simulink model "cps_stereo_analysis_v2"  (R2012b)
settings: Solver=FixedStepDiscrete  StartTime=0.0  StopTime=8.5  FixedStep=0.1  RelTol=1e-3  SampleTimeConstraint=STIndependent
libraries: visionutilities x3, visiongeotforms x3, visionstatistics x1, simulink x1
settings Model: RequirementInfo={} %GIDa_ba1ce617_85a9_495b_a3cb_2f0aceb7945f  MinMaxOverflowLogging=ForceOff  Creator=pmosterm  LastModifiedBy=pmosterm
settings SolverCC: EnableConcurrentExecution=on  ConcurrentTasks=on
settings DataIOCC: SignalLoggingSaveFormat=ModelDataLogs  SaveOutput=off  SaveTime=off
settings OptimizationCC: InlineParams=on
settings DebuggingCC: UnderspecifiedInitializationDetection=Simplified  FcnCallInpInsideContextMsg=EnableAllAsWarning  ModelReferenceExtraNoncontSigs=warning
settings ModelReferenceCC: ModelReferenceNumInstancesAllowed=Single
settings GRTTargetCC: CombineOutputUpdateFcns=off  GRTInterface=on
settings ConfigurationSet: Description=SimMechanics 2G

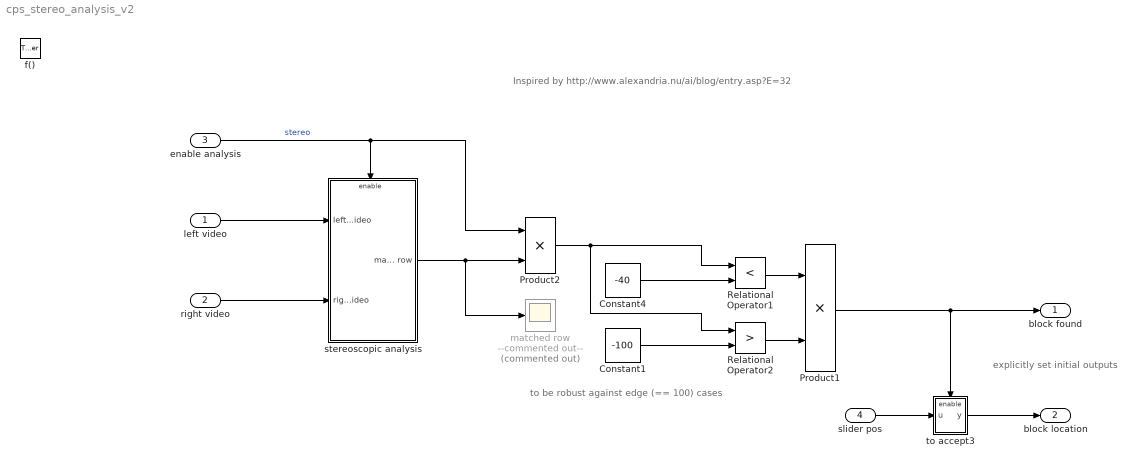
== system cps_stereo_analysis_v2 ==
  note: to be robust against
      | edge (== 100) cases
  note: Inspired by
      | http://www.alexandria.nu/ai/blog/entry.asp?E=32
  note: explicitly
      | set initial
      | outputs
  left video : Inport  OutDataTypeStr=uint8  PortDimensions=[400 240 3]
  right video : Inport  Port=2  OutDataTypeStr=uint8  PortDimensions=[400 240 3]
  enable analysis : Inport  Port=3  OutDataTypeStr=boolean  PortDimensions=1
  slider pos : Inport  Port=4  OutDataTypeStr=double  PortDimensions=1
  f() : TriggerPort  TriggerType=function-call  SampleTime=0.1  PortDimensions=1
  Constant1 : Constant  Value=-100  OutDataTypeStr=int16
  Constant4 : Constant  Value=-40  OutDataTypeStr=int16
  Product1 : Product  OutDataTypeStr=uint16  RndMeth=Zero
  Product2 : Product  RndMeth=Zero
  Relational Operator1 : RelationalOperator  Operator=<  OutDataTypeStr=fixdt(0,16)
  Relational Operator2 : RelationalOperator  Operator=>  OutDataTypeStr=fixdt(0,16)
  matched row --commented out-- : Scope  Commented=on
  stereoscopic analysis : Subsystem
  to accept3 : Subsystem  mask{yini=0}
      mask prompts: yini "Initial output"
      mask Display:
      | plot([1 2 3], [0 1 2]);
      | plot([1 2 3], [2 1 0]);
      | plot([5 6 7], [4 5 6]);
      | plot([5 6 7], [6 5 4]);
      | plot([9 10 11], [0 1 2]);
      | plot([9 10 11], [2 1 0]);
      | plot([0 6 6 12], [1 1 5 5]);
  block found : Outport  OutDataTypeStr=uint16  PortDimensions=1  InitialOutput=0
  block location : Outport  Port=2  OutDataTypeStr=double  PortDimensions=1  InitialOutput=0
  wires:
  left video/1 -> stereoscopic analysis/1(left video)
  enable analysis/1 -> Product2/1, stereoscopic analysis/Enable  "stereo"
  right video/1 -> stereoscopic analysis/2(right video)
  slider pos/1 -> to accept3/1(u)
  stereoscopic analysis/1(matched row) -> matched row --commented out--/1, Product2/2
  Constant4/1 -> Relational Operator1/2
  Product2/1 -> Relational Operator2/1, Relational Operator1/1
  to accept3/1(y) -> block location/1
  Constant1/1 -> Relational Operator2/2
  Relational Operator1/1 -> Product1/1
  Relational Operator2/1 -> Product1/2
  Product1/1 -> block found/1, to accept3/Enable

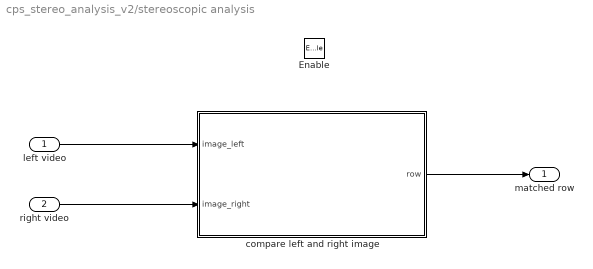
== system cps_stereo_analysis_v2/stereoscopic analysis ==
  left video : Inport
  right video : Inport  Port=2
  Enable : EnablePort
  compare left and right image : Subsystem  Variant=on  OverrideUsingVariant=textual
  matched row : Outport  InitialOutput=0
  wires:
  left video/1 -> compare left and right image/1(image_left)
  right video/1 -> compare left and right image/2(image_right)
  compare left and right image/1(row) -> matched row/1

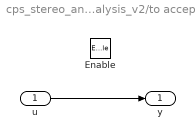
== system cps_stereo_analysis_v2/to accept3 ==
  u : Inport
  Enable : EnablePort
  y : Outport  InitialOutput=yini
  wires:
  u/1 -> y/1

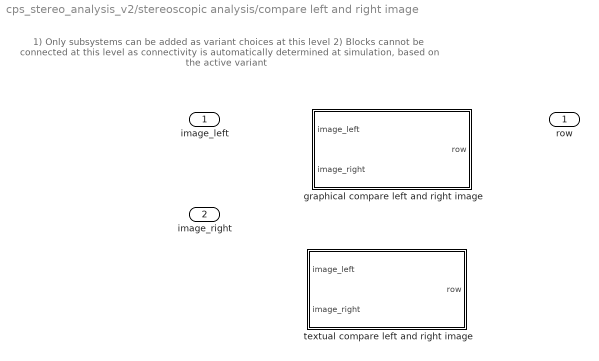
== system cps_stereo_analysis_v2/stereoscopic analysis/compare left and right image ==
  note: 1) Only subsystems can be added as variant choices at this level
      | 2) Blocks cannot be connected at this level as connectivity is
      | automatically determined at simulation, based on the active variant
  image_left : Inport
  image_right : Inport  Port=2
  graphical compare left and right image : Subsystem  VariantObject=graphical
  textual compare left and right image : MATLAB Function  TreatAsAtomicUnit=on  VariantObject=textual
  row : Outport

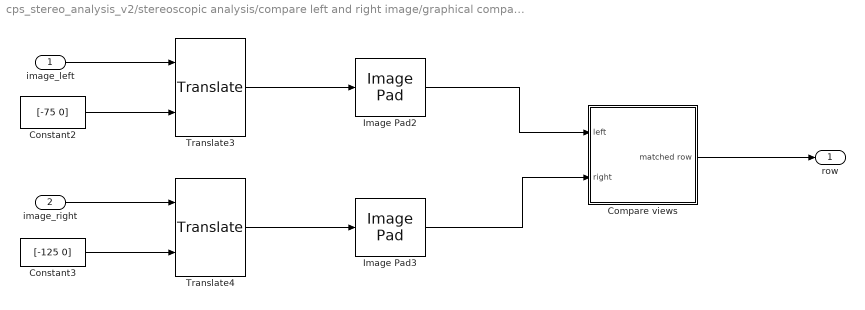
== system cps_stereo_analysis_v2/stereoscopic analysis/compare left and right image/graphical compare left and right image ==
  image_left : Inport
  image_right : Inport  Port=2
  Compare views : Subsystem  TreatAsAtomicUnit=on
  Constant2 : Constant  Value=[-75 0]  OutDataTypeStr=int16
  Constant3 : Constant  Value=[-125 0]  OutDataTypeStr=int16
  Image Pad2 : visionutilities/Image Pad  method=Constant  valSrc=Specify via dialog  value=0  spec=Output size  rowDirection=Right  outRowsMode=User-specified  rowSize=2  outColSize=120  colDirection=Bottom  outColsMode=User-specified  colSize=[60 80]  outRowSize=150  trunc_flag=None
  Image Pad3 : visionutilities/Image Pad  method=Constant  valSrc=Specify via dialog  value=0  spec=Output size  rowDirection=Right  outRowsMode=User-specified  rowSize=2  outColSize=120  colDirection=Bottom  outColsMode=User-specified  colSize=[60 80]  outRowSize=250  trunc_flag=None
  Translate3 : visiongeotforms/Translate  outSizeT=Same as input image  src_trans=Input port  translation="[1.5  2.3]"  maxOffset=[8 10]  fillVal=0  interpMethod=Bilinear  prodOutputMode=Binary point scaling  prodOutputWordLength=32  prodOutputFracLength=10  roundingMode=Nearest  overflowMode=on
  Translate4 : visiongeotforms/Translate  outSizeT=Same as input image  src_trans=Input port  translation="[1.5  2.3]"  maxOffset=[8 10]  fillVal=0  interpMethod=Bilinear  prodOutputMode=Binary point scaling  prodOutputWordLength=32  prodOutputFracLength=10  roundingMode=Nearest  overflowMode=on
  row : Outport
  wires:
  image_right/1 -> Translate4/1
  image_left/1 -> Translate3/1
  Constant2/1 -> Translate3/2
  Image Pad2/1 -> Compare views/1(left)
  Image Pad3/1 -> Compare views/2(right)
  Constant3/1 -> Translate4/2
  Translate3/1 -> Image Pad2/1
  Compare views/1(matched row) -> row/1
  Translate4/1 -> Image Pad3/1

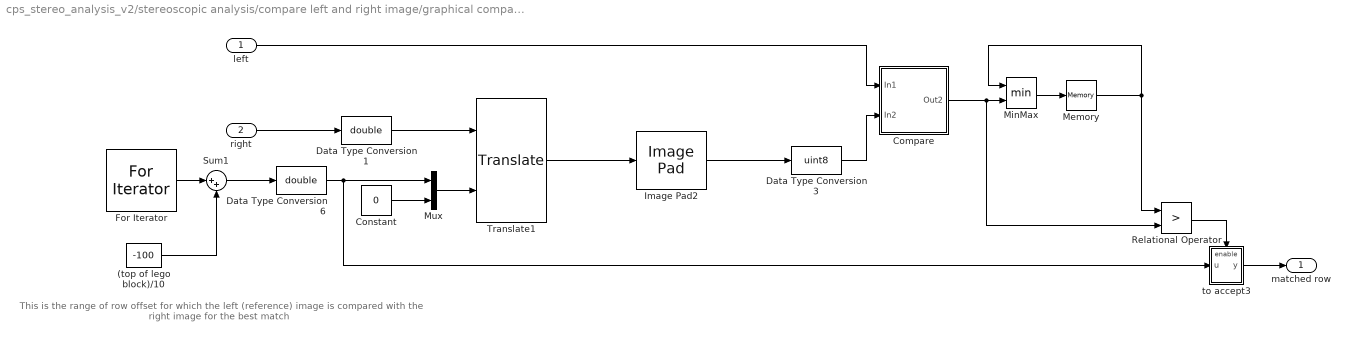
== system cps_stereo_analysis_v2/stereoscopic analysis/compare left and right image/graphical compare left and right image/Compare views ==
  note: This is the range of
      | row offset for which the
      | left (reference) image
      | is compared with the
      | right image for the
      | best match
  left : Inport
  right : Inport  Port=2
  (top of lego block)/10 : Constant  Value=-100
  Compare : Subsystem
  Constant : Constant  Value=0  OutDataTypeStr=double
  Data Type Conversion1 : DataTypeConversion  OutDataTypeStr=double
  Data Type Conversion3 : DataTypeConversion  OutDataTypeStr=uint8
  Data Type Conversion6 : DataTypeConversion  OutDataTypeStr=double
  For Iterator : ForIterator  ResetStates=reset  IterationLimit=100
  Image Pad2 : visionutilities/Image Pad  method=Constant  valSrc=Specify via dialog  value=0  spec=Output size  rowDirection=No padding  outRowsMode=User-specified  rowSize=2  outColSize=120  colDirection=Bottom  outColsMode=User-specified  colSize=[60 80]  outRowSize=150  trunc_flag=None
  Memory : Memory  X0=1e5  InheritSampleTime=on
  MinMax : MinMax  Inputs=2
  Mux : Mux  Inputs=2
  Relational Operator : RelationalOperator  Operator=>  OutDataTypeStr=boolean
  Sum1 : Sum  Inputs=|++
  Translate1 : visiongeotforms/Translate  outSizeT=Same as input image  src_trans=Input port  translation="[1.5  2.3]"  maxOffset=[8 10]  fillVal=0  interpMethod=Bilinear  prodOutputMode=Binary point scaling  prodOutputWordLength=32  prodOutputFracLength=10  roundingMode=Nearest  overflowMode=on
  to accept3 : Subsystem  mask{yini=0}
      mask prompts: yini "Initial output"
      mask Display:
      | plot([1 2 3], [0 1 2]);
      | plot([1 2 3], [2 1 0]);
      | plot([5 6 7], [4 5 6]);
      | plot([5 6 7], [6 5 4]);
      | plot([9 10 11], [0 1 2]);
      | plot([9 10 11], [2 1 0]);
      | plot([0 6 6 12], [1 1 5 5]);
  matched row : Outport  SourceOfInitialOutputValue=Input signal  InitialOutput=0
  wires:
  Data Type Conversion1/1 -> Translate1/1
  Data Type Conversion3/1 -> Compare/2(In2)
  left/1 -> Compare/1(In1)
  Sum1/1 -> Data Type Conversion6/1
  MinMax/1 -> Memory/1
  Compare/1(Out2) -> Relational Operator/2, MinMax/2
  right/1 -> Data Type Conversion1/1
  Constant/1 -> Mux/2
  Data Type Conversion6/1 -> Mux/1, to accept3/1(u)
  Mux/1 -> Translate1/2
  Image Pad2/1 -> Data Type Conversion3/1
  Memory/1 -> Relational Operator/1, MinMax/1
  Translate1/1 -> Image Pad2/1
  Relational Operator/1 -> to accept3/Enable
  to accept3/1(y) -> matched row/1
  For Iterator/1 -> Sum1/1
  (top of lego block)/10/1 -> Sum1/2

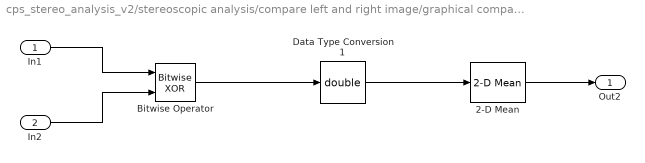
== system cps_stereo_analysis_v2/stereoscopic analysis/compare left and right image/graphical compare left and right image/Compare views/Compare ==
  In1 : Inport
  In2 : Inport  Port=2
  2-D Mean : visionstatistics/2-D Mean  run=off  reset_popup=None  directionMode=Entire input  dimension=1  treatSBRowAsCol=on  roiEnable=off  roiType=Rectangles  roiPortion=Entire ROI  roiOutput=Individual statistics for each ROI  roiFlag=off  outputDataTypeStr=Inherit: Same as accumulator  outputLastDataTypeStr=Inherit: Same as accumulator  outputMin=[]  outputMax=[]  accumMode=Binary point scaling  accumWordLength=32  accumFracLength=0  accumDataTypeStr=fixdt([],32,0)  accumLastDataTypeStr=fixdt([],32,0)  roundingMode=Floor  overflowMode=off
  Bitwise Operator : simulink/Logic and Bit Operations/Bitwise Operator  logicop=XOR  UseBitMask=off  NumInputPorts=2  BitMask=bin2dec('11011001')  BitMaskRealWorld=Stored Integer
  Data Type Conversion1 : DataTypeConversion  OutDataTypeStr=double  SaturateOnIntegerOverflow=on  RndMeth=Zero
  Out2 : Outport
  wires:
  Data Type Conversion1/1 -> 2-D Mean/1
  Bitwise Operator/1 -> Data Type Conversion1/1
  2-D Mean/1 -> Out2/1
  In1/1 -> Bitwise Operator/1
  In2/1 -> Bitwise Operator/2

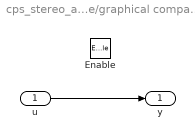
== system cps_stereo_analysis_v2/stereoscopic analysis/compare left and right image/graphical compare left and right image/Compare views/to accept3 ==
  u : Inport
  Enable : EnablePort
  y : Outport  InitialOutput=yini
  wires:
  u/1 -> y/1

== matlab function cps_stereo_analysis_v2/stereoscopic analysis/compare left and right image/textual compare left and right image ==
  data: image_left input; row output; image_right input
function row = fcn(image_left, image_right)
%#codegen

persistent hmean;
if isempty(hmean)
    hmean = video.Mean();
end

% number of successive image comparisons
nimages = 100;

% initialize the minimum mean and the corresponding row at which this mean
% is found for the number of successive image comparisons
min = 1e5;
row = 0;

% compute left image submatrix to successively compare
uint8_video_left = uint8(image_left);
left = uint8_video_left(75:224, 1:120, :);

% compute uint8 version of right image
uint8_video_right = uint8(image_right);

parfor k=1:nimages
    % compute successive right image submatrices for comparison
    right = uint8_video_right(125+k:125+149+k, 1:120, :);
    
    % compare left and right image submatrices
    cmp = bitxor(left,right);
    
    % compute the mean over all pixels of the comparison results
    pixel_mean = step(hmean,double(cmp));
    
    % in case of the final row only accept a substantially less
    % (at least 2) value of the mean
    if (pixel_mean < min && k < 100) || (pixel_mean < min - 2)
        min = pixel_mean;
        row = k;
    end
end

% to be consistent with negative offset in graphical version
row = - row;
